simulink model "AntilockBrake"  (R2020b)
settings: Solver=VariableStepAuto  StartTime=0.0  StopTime=10.0  RelTol=1e-3
settings Model: Creator=BIDITA PAUL  LastModifiedBy=BIDITA PAUL

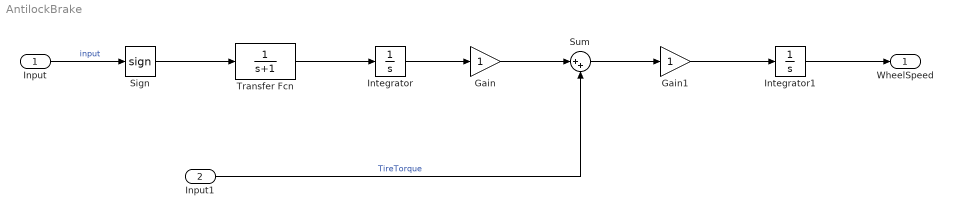
== system AntilockBrake ==
  Input : Inport
  Input1 : Inport  Port=2
  Gain : Gain
  Gain1 : Gain
  Integrator : Integrator
  Integrator1 : Integrator
  Sign : Signum
  Sum : Sum  Inputs=|++
  Transfer Fcn : TransferFcn  Denominator=[1 1]
  WheelSpeed : Outport
  wires:
  Sign/1 -> Transfer Fcn/1
  Transfer Fcn/1 -> Integrator/1
  Integrator/1 -> Gain/1
  Gain/1 -> Sum/1
  Sum/1 -> Gain1/1
  Gain1/1 -> Integrator1/1
  Input/1 -> Sign/1  "input"
  Input1/1 -> Sum/2  "TireTorque"
  Integrator1/1 -> WheelSpeed/1
